simulink model "SAR_ADC_2bit_CoSim_Analogue"  (R2024b)
settings: Solver=VariableStepAuto  StartTime=0.0  StopTime=0.908e-05  RelTol=1e-3
libraries: fl_lib x33, nesl_utility x8, ee_lib x4, simulink x4, msbDacArchitectures x2, fillib x1
settings Model: Creator=georg  LastModifiedBy=georg

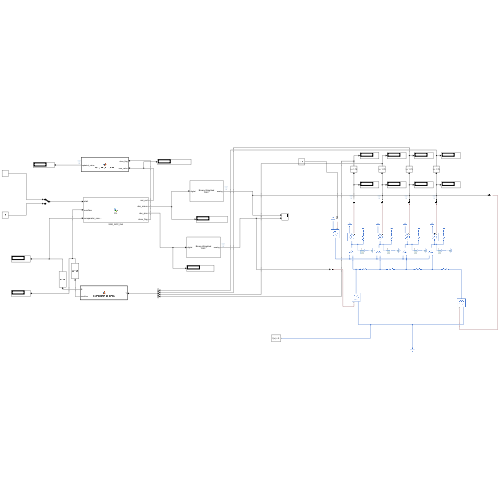
[thumbnail: Simulink's stored preview of the top-level diagram]
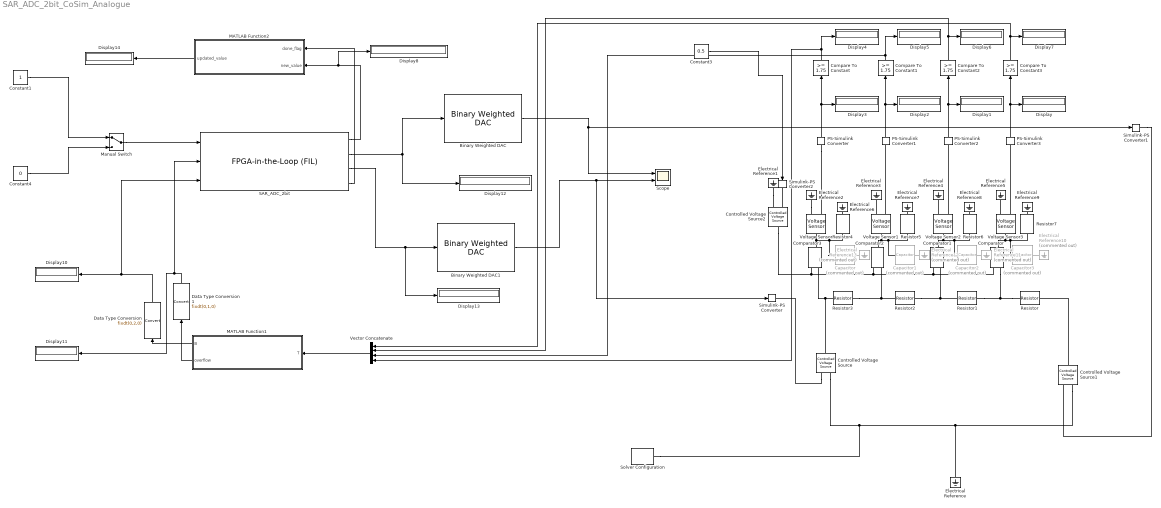
== system SAR_ADC_2bit_CoSim_Analogue ==
  Binary Weighted DAC : msbDacArchitectures/Binary Weighted DAC  NBits=16  Polarity=Unipolar  ExtStartClk=off  StartFreq=10e9  Ref=3.3  Bias=0  ReadySignal=off  EnableLinearityImpairments=on  OffsetError=0  OffsetErrorUnit=LSB  GainError=0  GainErrorUnit=LSB  EnableTimingImpairments=on  TimingSpecification=Settling time  SettlingTime=7.0618e-07  SettlingTimeTolerance=0.5  RisingSlewRate=2499994.5074  FallingSlewRate=-2499994.5074
  Binary Weighted DAC1 : msbDacArchitectures/Binary Weighted DAC  NBits=16  Polarity=Unipolar  ExtStartClk=off  StartFreq=10e09  Ref=3.3  Bias=0  ReadySignal=off  EnableLinearityImpairments=on  OffsetError=0  OffsetErrorUnit=LSB  GainError=0  GainErrorUnit=LSB  EnableTimingImpairments=on  TimingSpecification=Slew rate  SettlingTime=7.0618e-07  SettlingTimeTolerance=0.5  RisingSlewRate=2.5e6  FallingSlewRate=-2.5e6
  Capacitor{,1..3} (4 alike) : fl_lib/Electrical/Electrical Elements/Capacitor  Commented=on  c=10 nF  r=1e-6 Ohm  g=0 1/Ohm  i_specify=off  i_priority=None  i=0 A  i_nominal_specify=off  i_nominal_value=1  i_nominal_unit=A  v_specify=off  v_priority=None  v=0 V  v_nominal_specify=off  v_nominal_value=1  v_nominal_unit=V  vc_specify=off  vc_priority=High  vc=0 V  vc_nominal_specify=off  vc_nominal_value=1  vc_nominal_unit=V
  Comparator : ee_lib/Integrated Circuits/Comparator  V_OS=5 mV  C_IN=2.5 pF  V_OL=0 V  V_OH=3.3 V  R_OUT=100 Ohm  Delay=300 ns
      settings: InternalSimscapePortConfiguration="{\"Bottom\":[],\"Left\":[{\"id\":\"p\",\"label\":\"+\",\"type\":\"foundation.electrical.electrical\"},{\"id\":\"n\",\"label\":\"-\",\"type\":\"foundation.electrical.electrical\"}],\"Right\":[{\"id\":\"J\",\"label\":\"\",\"type\":\"foundation.electrical.electrical\"}],\"Top\":[]}"
  Comparator1 : ee_lib/Integrated Circuits/Comparator  V_OS=5 mV  C_IN=2.5 pF  V_OL=0 V  V_OH=3.3 V  R_OUT=100 Ohm  Delay=300 ns
      settings: InternalSimscapePortConfiguration="{\"Bottom\":[],\"Left\":[{\"id\":\"p\",\"label\":\"+\",\"type\":\"foundation.electrical.electrical\"},{\"id\":\"n\",\"label\":\"-\",\"type\":\"foundation.electrical.electrical\"}],\"Right\":[{\"id\":\"J\",\"label\":\"\",\"type\":\"foundation.electrical.electrical\"}],\"Top\":[]}"
  Comparator2 : ee_lib/Integrated Circuits/Comparator  V_OS=5 mV  C_IN=2.5 pF  V_OL=0 V  V_OH=3.3 V  R_OUT=100 Ohm  Delay=300 ns
      settings: InternalSimscapePortConfiguration="{\"Bottom\":[],\"Left\":[{\"id\":\"p\",\"label\":\"+\",\"type\":\"foundation.electrical.electrical\"},{\"id\":\"n\",\"label\":\"-\",\"type\":\"foundation.electrical.electrical\"}],\"Right\":[{\"id\":\"J\",\"label\":\"\",\"type\":\"foundation.electrical.electrical\"}],\"Top\":[]}"
  Comparator3 : ee_lib/Integrated Circuits/Comparator  V_OS=0.5 mV  C_IN=2.5 pF  V_OL=0 V  V_OH=3.3 V  R_OUT=100 Ohm  Delay=300 ns
      settings: InternalSimscapePortConfiguration="{\"Bottom\":[],\"Left\":[{\"id\":\"p\",\"label\":\"+\",\"type\":\"foundation.electrical.electrical\"},{\"id\":\"n\",\"label\":\"-\",\"type\":\"foundation.electrical.electrical\"}],\"Right\":[{\"id\":\"J\",\"label\":\"\",\"type\":\"foundation.electrical.electrical\"}],\"Top\":[]}"
  Compare To Constant{,1..3} (4 alike) : simulink/Logic and Bit Operations/Compare To Constant  relop=>=  const=1.75  OutDataTypeStr=boolean
  Constant1 : Constant  VectorParams1D=off  OutDataTypeStr=fixdt(0,1,0, 'DataTypeOverride', 'Off')  SampleTime=-1
  Constant3 : Constant  Value=0.5
  Constant4 : Constant  Value=0  VectorParams1D=off  OutDataTypeStr=fixdt(0,1,0)  SampleTime=-1
  Controlled Voltage Source : fl_lib/Electrical/Electrical Sources/Controlled Voltage Source
  Controlled Voltage Source1 : fl_lib/Electrical/Electrical Sources/Controlled Voltage Source
  Controlled Voltage Source2 : fl_lib/Electrical/Electrical Sources/Controlled Voltage Source
  Data Type Conversion : DataTypeConversion  OutDataTypeStr=fixdt(0,2,0)  SaturateOnIntegerOverflow=off  RndMeth=Floor
  Data Type Conversion1 : DataTypeConversion  OutDataTypeStr=fixdt(0,1,0)  SaturateOnIntegerOverflow=off  RndMeth=Floor
  Display{,1..8,10..14} (14 alike) : Display
      Display10 settings: Format=binary (Stored Integer)
      Display11 settings: Format=binary (Stored Integer)
      Display12 settings: Format=binary (Stored Integer)
      Display13 settings: Format=binary (Stored Integer)
      Display14 settings: Format=binary (Stored Integer)  Decimation=2
      Display8 settings: Format=binary (Stored Integer)
  Electrical Reference{,1..9} (10 alike) : fl_lib/Electrical/Electrical Elements/Electrical Reference
  Electrical Reference{10..13} (4 alike) : fl_lib/Electrical/Electrical Elements/Electrical Reference  Commented=on
  MATLAB Function1 : MATLAB Function  TreatAsAtomicUnit=on  SystemSampleTime=1e-08
  MATLAB Function2 : MATLAB Function  TreatAsAtomicUnit=on  SystemSampleTime=1e-08
  Manual Switch : ManualSwitch
  PS-Simulink Converter{,1..3} (4 alike) : nesl_utility/PS-Simulink Converter  PhysicalDomain=network_engine_domain  SubClassName=ps_output  LeftPortType=input  RightPortType=output  PseudoPeriodic=off  Frequencies=[]  VectorFormat=inherit  Unit=inherit  AffineConversion=off
  Resistor{,1..3} (4 alike) : fl_lib/Electrical/Electrical Elements/Resistor  R=1 kOhm  i_specify=off  i_priority=None  i=0 A  i_nominal_specify=off  i_nominal_value=1  i_nominal_unit=A  v_specify=off  v_priority=None  v=0 V  v_nominal_specify=off  v_nominal_value=1  v_nominal_unit=V
  Resistor{4..7} (4 alike) : fl_lib/Electrical/Electrical Elements/Resistor  R=10 MOhm  i_specify=off  i_priority=None  i=0 A  i_nominal_specify=off  i_nominal_value=1  i_nominal_unit=A  v_specify=off  v_priority=None  v=0 V  v_nominal_specify=off  v_nominal_value=1  v_nominal_unit=V
  SAR_ADC_2bit : fillib/FPGA-in-the-Loop (FIL)  ForceInterfaceUpdate=0.09754
  Scope : Scope  NumInputPorts=2
  Simulink-PS Converter : nesl_utility/Simulink-PS Converter  PhysicalDomain=network_engine_domain  SubClassName=ps_input  LeftPortType=input  RightPortType=output  PseudoPeriodic=off  Frequencies=[]  NoiseDistribution=none  NoiseParameters=[]  Unit=V  AffineConversion=off  FilteringAndDerivatives=provide  SimscapeFilterOrder=1  InputFilterTimeConstant=0.001  UdotUserProvided=0
  Simulink-PS Converter1 : nesl_utility/Simulink-PS Converter  PhysicalDomain=network_engine_domain  SubClassName=ps_input  LeftPortType=input  RightPortType=output  PseudoPeriodic=off  Frequencies=[]  NoiseDistribution=none  NoiseParameters=[]  Unit=V  AffineConversion=off  FilteringAndDerivatives=provide  SimscapeFilterOrder=1  InputFilterTimeConstant=0.001  UdotUserProvided=0
  Simulink-PS Converter2 : nesl_utility/Simulink-PS Converter  PhysicalDomain=network_engine_domain  SubClassName=ps_input  LeftPortType=input  RightPortType=output  PseudoPeriodic=off  Frequencies=[]  NoiseDistribution=none  NoiseParameters=[]  Unit=V  AffineConversion=off  FilteringAndDerivatives=provide  SimscapeFilterOrder=1  InputFilterTimeConstant=0.001  UdotUserProvided=0
  Solver Configuration : nesl_utility/Solver Configuration  PhysicalDomain=network_engine_domain  SubClassName=solver  LeftPortType=input  RightPortType=generic  Tones=[]  Harmonics=[]  SimulateNoise=off  Profile=off  UseLocalSampling=off  EnableSwitchedLinearOptims=on  FrequencyDomain=off  UseCCode=off  RelTol=0.001  AbsTol=0.001  MinStep=1e-09  ToWorkspace=off  RevertToSquareIcSolve=off  NumHomotopyIterations=100  PhasorMode=off  PhasorModeNumHarmonics=1  ConsistencySolver=NEWTON_XTOL_AFTER_FTOL  IndexReductionMethod=DerivativeReplacement  DoDC=off  ResidualTolerance=1e-09  ConsistencyTolSource=GLOBAL  ConsistencyAbsTol=0.001  ConsistencyRelTol=0.001  ConsistencyTolFactor=0.001  UseLocalSolver=off  LocalSolverChoice=NE_BACKWARD_EULER_ADVANCER  ResolveIndetEquations=on  FunctionEvalNumThread=1  LocalSolverSampleTime=0.001  DoFixedCost=off  MaxNonlinIter=3  MaxModeIter=2  ComputeImpulses=off  ImpulseIterations=2  LinearAlgebra=auto  LinearAlgebraNumThread=0  EquationFormulation=NE_TIME_EF  DelaysMemoryBudget=1024  AutomaticFiltering=on  FilteringTimeConstant=0.001  PartitionStorageMethod=AS_NEEDED  PartitionMemoryBudget=1024  PartitionMethod=ROBUST  MultibodyUseLocalSolver=off  MultibodyLocalSolverChoice=ODE1  MultibodyLocalSolverSampleTime=0.001
  Vector Concatenate : Concatenate  NumInputs=4
  Voltage Sensor{,1..3} (4 alike) : fl_lib/Electrical/Electrical Sensors/Voltage Sensor
  wires:
  Constant3/1 -> Simulink-PS Converter2/1
  PS-Simulink Converter/1 -> Compare To Constant/1, Display3/1
  PS-Simulink Converter1/1 -> Compare To Constant1/1, Display2/1
  PS-Simulink Converter2/1 -> Compare To Constant2/1, Display1/1
  PS-Simulink Converter3/1 -> Compare To Constant3/1, Display/1
  Compare To Constant3/1 -> Vector Concatenate/1, Display7/1
  Compare To Constant2/1 -> Display6/1, Vector Concatenate/2
  Compare To Constant1/1 -> Display5/1, Vector Concatenate/3
  Compare To Constant/1 -> Display4/1, Vector Concatenate/4
  MATLAB Function1/2(overflow) -> Data Type Conversion1/1
  Data Type Conversion/1 -> SAR_ADC_2bit/3, Display10/1
  MATLAB Function2/1(updated_value) -> Display14/1
  Constant4/1 -> Manual Switch/2
  Constant1/1 -> Manual Switch/1
  Binary Weighted DAC1/1 -> Simulink-PS Converter/1, Scope/2
  MATLAB Function1/1(B) -> Data Type Conversion/1
  Data Type Conversion1/1 -> SAR_ADC_2bit/2, Display11/1
  Binary Weighted DAC/1 -> Simulink-PS Converter1/1, Scope/1
  Vector Concatenate/1 -> MATLAB Function1/1(T)
  Manual Switch/1 -> SAR_ADC_2bit/1
  SAR_ADC_2bit/1 -> Display8/1, MATLAB Function2/2(new_value)
  SAR_ADC_2bit/2 -> Display12/1, Binary Weighted DAC/1
  SAR_ADC_2bit/3 -> Display13/1, Binary Weighted DAC1/1
  SAR_ADC_2bit/4 -> MATLAB Function2/1(done_flag)
  connections:
  Resistor3/LConn1 -- Comparator3/LConn2 -- Controlled Voltage Source/LConn1
  Resistor/LConn1 -- Resistor1/RConn1 -- Comparator/LConn2
  Resistor2/RConn1 -- Resistor1/LConn1 -- Comparator1/LConn2
  Resistor3/RConn1 -- Resistor2/LConn1 -- Comparator2/LConn2
  Controlled Voltage Source/RConn2 -- Solver Configuration/RConn1 -- Controlled Voltage Source1/RConn2 -- Electrical Reference/LConn1
  Comparator3/LConn1 -- Controlled Voltage Source2/LConn1 -- Comparator/LConn1 -- Comparator1/LConn1 -- Comparator2/LConn1
  Controlled Voltage Source2/RConn1 -- Simulink-PS Converter2/RConn1
  Controlled Voltage Source1/LConn1 -- Resistor/RConn1
  Simulink-PS Converter1/RConn1 -- Controlled Voltage Source1/RConn1
  Electrical Reference1/LConn1 -- Controlled Voltage Source2/RConn2
  Controlled Voltage Source/RConn1 -- Simulink-PS Converter/RConn1
  Voltage Sensor/LConn1 -- Capacitor/LConn1 -- Resistor4/LConn1 -- Comparator3/RConn1
  Voltage Sensor1/LConn1 -- Comparator2/RConn1 -- Resistor5/LConn1 -- Capacitor1/LConn1
  Voltage Sensor2/LConn1 -- Comparator1/RConn1 -- Capacitor2/LConn1 -- Resistor6/LConn1
  Voltage Sensor3/LConn1 -- Comparator/RConn1 -- Capacitor3/LConn1 -- Resistor7/LConn1
  Electrical Reference2/LConn1 -- Voltage Sensor/RConn2
  Voltage Sensor1/RConn2 -- Electrical Reference3/LConn1
  Voltage Sensor2/RConn2 -- Electrical Reference4/LConn1
  Voltage Sensor3/RConn2 -- Electrical Reference5/LConn1
  PS-Simulink Converter/LConn1 -- Voltage Sensor/RConn1
  Voltage Sensor1/RConn1 -- PS-Simulink Converter1/LConn1
  Voltage Sensor2/RConn1 -- PS-Simulink Converter2/LConn1
  Voltage Sensor3/RConn1 -- PS-Simulink Converter3/LConn1
  Electrical Reference6/LConn1 -- Resistor4/RConn1
  Electrical Reference7/LConn1 -- Resistor5/RConn1
  Electrical Reference8/LConn1 -- Resistor6/RConn1
  Electrical Reference9/LConn1 -- Resistor7/RConn1
  Electrical Reference10/LConn1 -- Capacitor3/RConn1
  Electrical Reference11/LConn1 -- Capacitor2/RConn1
  Electrical Reference12/LConn1 -- Capacitor1/RConn1
  Electrical Reference13/LConn1 -- Capacitor/RConn1

== matlab function SAR_ADC_2bit_CoSim_Analogue/MATLAB Function2 ==
  data: done_flag input; new_value input; updated_value output
function updated_value = rising_edge_update(done_flag, new_value)
    %#codegen
    % Ensure input types are properly handled
    done_flag = double(done_flag); % Convert fixed-point to double
    new_value = double(new_value); % Ensure new_value is also double

    % Persistent variables
    persistent prev_done_flag output_value

    if isempty(prev_done_flag)
        prev_done_flag = 0;    % Initialize as double
        output_value = 0;      % Initialize output value as double
    end
    
    % Rising edge detection
    if done_flag == 1 && prev_done_flag == 0
        output_value = new_value; % Update value only on rising edge
    end
    
    % Store previous state
    prev_done_flag = done_flag;
    
    % Output result as double
    updated_value = output_value*(3.3/(2^16 -1));
end


%*(3.3/(2^16 -1))

== matlab function SAR_ADC_2bit_CoSim_Analogue/MATLAB Function1 ==
  data: T input; B output; overflow output
function [B, overflow] = thermometer_to_binary(T)
    % Converts 4-bit thermometer code to a 2-bit binary output and overflow flag.

    % Ensure T is a row vector
    T = T(:)'; 

    % Convert thermometer code to binary value
    bin_val = sum(T);
    overflow_int =0;
    
    % Set overflow flag if all bits are 1
    if bin_val == 4
        overflow_int = 1;
        bin_val = 3;
    end
    % Convert bin_val to a 2-bit binary number
    B = uint8(bin_val);
    overflow = overflow_int;

end
